simulink model "ClosedLoopPMSM"  (R2019a)
settings: Solver=FixedStepAuto  StartTime=0.0  StopTime=inf  FixedStep=Sampling_time  RelTol=1e-3
values from neighbouring files (symbols this model uses):
  DCLINK_Cap = 100e-6    (= 0.0001)    [ClosedLoopParameters.m]
  interleaving_angle_1 = 0    [ClosedLoopParameters.m]
  Rin = 1e-6    (= 1e-06)    [ClosedLoopParameters.m]
  Sampling_time = 1e-6    (= 1e-06)    [ClosedLoopParameters.m]
  Vin = Vdesired    (= 540)    [ClosedLoopParameters.m]
undefined symbols (not defined in the file or in its folder): Tload
libraries: powerlib x7, eeTransforms x4, simulink x3, powerlib_meascontrol x1
settings Model: Creator=admin  LastModifiedBy=admin

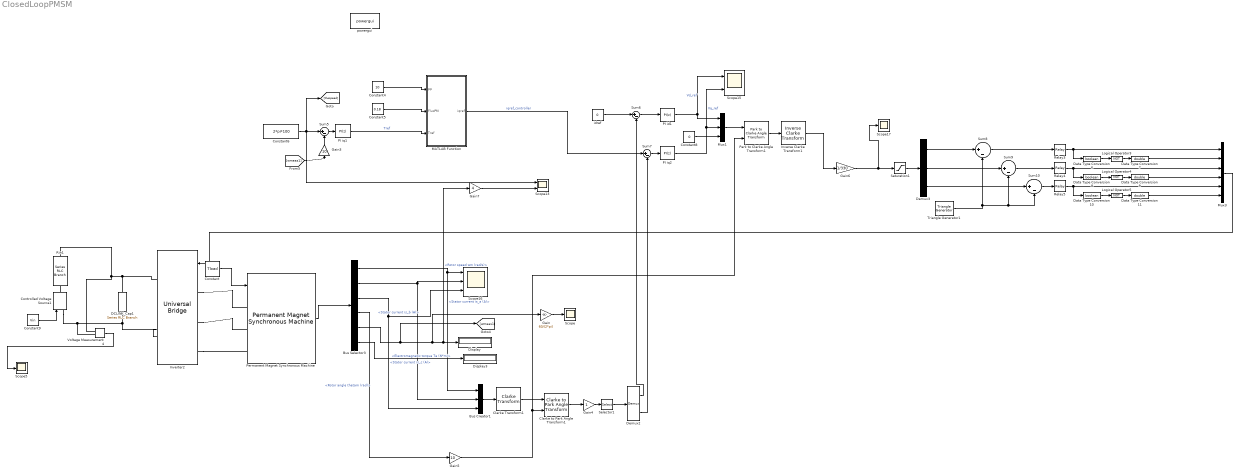
== system ClosedLoopPMSM ==
  Bus Creator1 : BusCreator  Inputs=3
  Bus Selector3 : BusSelector  OutputSignals=Stator current is_a (A),Stator current is_b (A),Stator current is_c (A),Rotor angle thetam (rad),Rotor speed wm (rad/s),Electromagnetic torque Te (N*m)
  Clarke Transform1 : eeTransforms/Clarke Transform  PowerInvariant=off
      settings: SourceProductName=Simscape Electrical  SourceProductBaseCode=PS
  Clarke to Park Angle Transform1 : eeTransforms/Clarke to Park Angle Transform  AxisAlignment=Q-axis
      settings: SourceProductName=Simscape Electrical  SourceProductBaseCode=PS
  Constant : Constant  Value=Tload
  Constant4 : Constant  Value=10
  Constant5 : Constant  Value=0.18
  Constant6 : Constant  Value=2*pi*100
  Constant8 : Constant  Value=0
  Constant9 : Constant  Value=Vin
  Controlled Voltage Source1 : powerlib/Electrical Sources/Controlled Voltage Source  Initialize=on  Source_Type=DC  Amplitude=0  Phase=0  Frequency=0  Measurements=None
      settings: SourceProductName=Simscape Electrical
  DCLINK_Cap1 : powerlib/Elements/Series RLC Branch  LConnTagsString=__new0  RConnTagsString=__new0  BranchType=C  Resistance=1  Inductance=1e-3  SetiL0=off  InitialCurrent=0  Capacitance=DCLINK_Cap  Setx0=on  InitialVoltage=540  Measurements=None
      settings: SourceProductName=Simscape Electrical
  Data Type Conversion10 : DataTypeConversion  OutDataTypeStr=boolean
  Data Type Conversion11 : DataTypeConversion  OutDataTypeStr=double
  Data Type Conversion6 : DataTypeConversion  OutDataTypeStr=boolean
  Data Type Conversion7 : DataTypeConversion  OutDataTypeStr=double
  Data Type Conversion8 : DataTypeConversion  OutDataTypeStr=boolean
  Data Type Conversion9 : DataTypeConversion  OutDataTypeStr=double
  Demux2 : Demux  Outputs=2
  Demux3 : Demux  Outputs=3
  Display : Display
  Display3 : Display
  Gain : Gain  Gain=60/(2*pi)
  Gain3 : Gain  Gain=10
  Gain4 : Gain
  Gain5 : Gain  Gain=10
  Gain6 : Gain  Gain=1/330
  Gain7 : Gain  Gain=4
  Inverse Clarke Transform1 : eeTransforms/Inverse Clarke Transform  PowerInvariant=off
      settings: SourceProductName=Simscape Electrical  SourceProductBaseCode=PS
  Inverter2 : powerlib/Power Electronics/Universal Bridge  Arms=3  SnubberResistance=1e5  SnubberCapacitance=inf  Device=IGBT / Diodes  Ron=0.65e-3  Lon=0  ForwardVoltages="[  0  0  ]"  ForwardVoltage=0  GTOparameters=[ 10e-6 , 20e-6 ]  IGBTparameters=[ 1e-6 , 2e-6 ]  Measurements=All voltages and currents  Measurements_2=None  converterType=Rectifier
      settings: SourceProductName=Simscape Electrical
  Logical Operator3 : Logic  Operator=NOT  AllPortsSameDT=off  OutDataTypeStr=boolean
  Logical Operator4 : Logic  Operator=NOT  AllPortsSameDT=off  OutDataTypeStr=boolean
  Logical Operator5 : Logic  Operator=NOT  AllPortsSameDT=off  OutDataTypeStr=boolean
  MATLAB Function : MATLAB Function  TreatAsAtomicUnit=on
  Mux1 : Mux  Inputs=3
  Mux3 : Mux  Inputs=6
  PI id1 : simulink/Continuous/PID Controller  Controller=PI  Form=Parallel  TimeDomain=Discrete-time  SampleTime=-1  IntegratorMethod=Forward Euler  FilterMethod=Forward Euler  ControllerParametersSource=internal  P=0.5  I=5  D=0  UseFilter=on  N=100  TunerSelectOption=Transfer Function Based (PID Tuner App)  InitialConditionSource=internal  InitialConditionForIntegrator=0  InitialConditionForFilter=0  DifferentiatorICPrevScaledInput=0  ExternalReset=none  TrackingMode=off  Kt=1  LimitOutput=off  UpperSaturationLimit=inf  LowerSaturationLimit=-inf  LinearizeAsGain=on  AntiWindupMode=none  Kb=1  POutMin=[]  POutMax=[]  IOutMin=[]  IOutMax=[]  DOutMin=[]  DOutMax=[]  NOutMin=[]  NOutMax=[]  SumOutMin=[]  SumOutMax=[]  SaturationOutMin=[]  SaturationOutMax=[]  PParamMin=[]  PParamMax=[]  IParamMin=[]  IParamMax=[]  DParamMin=[]  DParamMax=[]  NParamMin=[]  NParamMax=[]  KbParamMin=[]  KbParamMax=[]  KtParamMin=[]  KtParamMax=[]  KbOutMin=[]  KbOutMax=[]  KtOutMin=[]  KtOutMax=[]  IntegratorOutMin=[]  IntegratorOutMax=[]  FilterOutMin=[]  FilterOutMax=[]  SumI1OutMin=[]  SumI1OutMax=[]  SumI2OutMin=[]  SumI2OutMax=[]  SumI3OutMin=[]  SumI3OutMax=[]  SumI4OutMin=[]  SumI4OutMax=[]  SumDOutMin=[]  SumDOutMax=[]  DifferentiatorOutMin=[]  DifferentiatorOutMax=[]  FilterDiffOutCoefMin=[]  FilterDiffOutCoefMax=[]  ReciprocalOutMin=[]  ReciprocalOutMax=[]  SumDenOutMin=[]  SumDenOutMax=[]  SumNumOutMin=[]  SumNumOutMax=[]  DivideOutMin=[]  DivideOutMax=[]  IntegratorContinuousStateAttributes=''  IntegratorStateMustResolveToSignalObject=off  IntegratorRTWStateStorageClass=Auto  FilterContinuousStateAttributes=''  FilterStateMustResolveToSignalObject=off  FilterRTWStateStorageClass=Auto  ParallelPVariant=InternalParameters  IdealPVariant=Disabled  IVariant=InternalParameters  DVariant=Disabled  IntegratorVariant=Discrete  SatVariant=Disabled  AWVariant=Passthrough  PCopyVariant=Disabled  TRVariant=Disabled  FdbkBlocksVariant=Forward  IdealPFdbkVariant=Disabled  SatFdbkVariant=Disabled  DerivativeFilterVariant=Disabled  NVariant=Disabled  NCopyVariant=Disabled_SignalSpec  FilterICVariant=Disabled  IntegratorICVariant=InternalICs  ExternalResetVariant=Disabled  TRSumVariant=Passthrough  SumFdbkVariant=Disabled  SumVariant=Sum_PI
  PI iq1 : simulink/Continuous/PID Controller  Controller=PI  Form=Parallel  TimeDomain=Discrete-time  SampleTime=-1  IntegratorMethod=Forward Euler  FilterMethod=Forward Euler  ControllerParametersSource=internal  P=100  I=10  D=0  UseFilter=on  N=100  TunerSelectOption=Transfer Function Based (PID Tuner App)  InitialConditionSource=internal  InitialConditionForIntegrator=0  InitialConditionForFilter=0  DifferentiatorICPrevScaledInput=0  ExternalReset=none  TrackingMode=off  Kt=1  LimitOutput=off  UpperSaturationLimit=inf  LowerSaturationLimit=-inf  LinearizeAsGain=on  AntiWindupMode=none  Kb=1  POutMin=[]  POutMax=[]  IOutMin=[]  IOutMax=[]  DOutMin=[]  DOutMax=[]  NOutMin=[]  NOutMax=[]  SumOutMin=[]  SumOutMax=[]  SaturationOutMin=[]  SaturationOutMax=[]  PParamMin=[]  PParamMax=[]  IParamMin=[]  IParamMax=[]  DParamMin=[]  DParamMax=[]  NParamMin=[]  NParamMax=[]  KbParamMin=[]  KbParamMax=[]  KtParamMin=[]  KtParamMax=[]  KbOutMin=[]  KbOutMax=[]  KtOutMin=[]  KtOutMax=[]  IntegratorOutMin=[]  IntegratorOutMax=[]  FilterOutMin=[]  FilterOutMax=[]  SumI1OutMin=[]  SumI1OutMax=[]  SumI2OutMin=[]  SumI2OutMax=[]  SumI3OutMin=[]  SumI3OutMax=[]  SumI4OutMin=[]  SumI4OutMax=[]  SumDOutMin=[]  SumDOutMax=[]  DifferentiatorOutMin=[]  DifferentiatorOutMax=[]  FilterDiffOutCoefMin=[]  FilterDiffOutCoefMax=[]  ReciprocalOutMin=[]  ReciprocalOutMax=[]  SumDenOutMin=[]  SumDenOutMax=[]  SumNumOutMin=[]  SumNumOutMax=[]  DivideOutMin=[]  DivideOutMax=[]  IntegratorContinuousStateAttributes=''  IntegratorStateMustResolveToSignalObject=off  IntegratorRTWStateStorageClass=Auto  FilterContinuousStateAttributes=''  FilterStateMustResolveToSignalObject=off  FilterRTWStateStorageClass=Auto  ParallelPVariant=InternalParameters  IdealPVariant=Disabled  IVariant=InternalParameters  DVariant=Disabled  IntegratorVariant=Discrete  SatVariant=Disabled  AWVariant=Passthrough  PCopyVariant=Disabled  TRVariant=Disabled  FdbkBlocksVariant=Forward  IdealPFdbkVariant=Disabled  SatFdbkVariant=Disabled  DerivativeFilterVariant=Disabled  NVariant=Disabled  NCopyVariant=Disabled_SignalSpec  FilterICVariant=Disabled  IntegratorICVariant=InternalICs  ExternalResetVariant=Disabled  TRSumVariant=Passthrough  SumFdbkVariant=Disabled  SumVariant=Sum_PI
  PI iq2 : simulink/Continuous/PID Controller  Controller=PI  Form=Parallel  TimeDomain=Discrete-time  SampleTime=-1  IntegratorMethod=Forward Euler  FilterMethod=Forward Euler  ControllerParametersSource=internal  P=0.5  I=5  D=0  UseFilter=on  N=100  TunerSelectOption=Transfer Function Based (PID Tuner App)  InitialConditionSource=internal  InitialConditionForIntegrator=0  InitialConditionForFilter=0  DifferentiatorICPrevScaledInput=0  ExternalReset=none  TrackingMode=off  Kt=1  LimitOutput=off  UpperSaturationLimit=inf  LowerSaturationLimit=-inf  LinearizeAsGain=on  AntiWindupMode=none  Kb=1  POutMin=[]  POutMax=[]  IOutMin=[]  IOutMax=[]  DOutMin=[]  DOutMax=[]  NOutMin=[]  NOutMax=[]  SumOutMin=[]  SumOutMax=[]  SaturationOutMin=[]  SaturationOutMax=[]  PParamMin=[]  PParamMax=[]  IParamMin=[]  IParamMax=[]  DParamMin=[]  DParamMax=[]  NParamMin=[]  NParamMax=[]  KbParamMin=[]  KbParamMax=[]  KtParamMin=[]  KtParamMax=[]  KbOutMin=[]  KbOutMax=[]  KtOutMin=[]  KtOutMax=[]  IntegratorOutMin=[]  IntegratorOutMax=[]  FilterOutMin=[]  FilterOutMax=[]  SumI1OutMin=[]  SumI1OutMax=[]  SumI2OutMin=[]  SumI2OutMax=[]  SumI3OutMin=[]  SumI3OutMax=[]  SumI4OutMin=[]  SumI4OutMax=[]  SumDOutMin=[]  SumDOutMax=[]  DifferentiatorOutMin=[]  DifferentiatorOutMax=[]  FilterDiffOutCoefMin=[]  FilterDiffOutCoefMax=[]  ReciprocalOutMin=[]  ReciprocalOutMax=[]  SumDenOutMin=[]  SumDenOutMax=[]  SumNumOutMin=[]  SumNumOutMax=[]  DivideOutMin=[]  DivideOutMax=[]  IntegratorContinuousStateAttributes=''  IntegratorStateMustResolveToSignalObject=off  IntegratorRTWStateStorageClass=Auto  FilterContinuousStateAttributes=''  FilterStateMustResolveToSignalObject=off  FilterRTWStateStorageClass=Auto  ParallelPVariant=InternalParameters  IdealPVariant=Disabled  IVariant=InternalParameters  DVariant=Disabled  IntegratorVariant=Discrete  SatVariant=Disabled  AWVariant=Passthrough  PCopyVariant=Disabled  TRVariant=Disabled  FdbkBlocksVariant=Forward  IdealPFdbkVariant=Disabled  SatFdbkVariant=Disabled  DerivativeFilterVariant=Disabled  NVariant=Disabled  NCopyVariant=Disabled_SignalSpec  FilterICVariant=Disabled  IntegratorICVariant=InternalICs  ExternalResetVariant=Disabled  TRSumVariant=Passthrough  SumFdbkVariant=Disabled  SumVariant=Sum_PI
  Park to Clarke Angle Transform1 : eeTransforms/Park to Clarke Angle Transform  AxisAlignment=Q-axis
      settings: SourceProductName=Simscape Electrical  SourceProductBaseCode=PS
  Permanent Magnet Synchronous Machine : powerlib/Machines/Permanent Magnet Synchronous Machine  NbPhases=3  FluxDistribution=Sinusoidal  RotorType=Salient-pole  MechanicalLoad=Torque Tm  PresetModel=No  ShowDetailedParameters=on  MeasurementBus=off  Resistance=0.320  Inductance=8.5e-3  dqInductances=[3.1e-3,3.6e-3]  La=0.000395  MachineConstant=Flux linkage established by magnets (V.s)  Flux=0.18  VoltageCst=326.4839  TorqueCst=2.7  Flat=120  Mechanical=[0.0027 0.0004924 10 0]  PolePairs=4  InitialConditions=[0,0, 0,0]  InitialConditions5ph=[0 0 0 0 0 0]  TsPowergui=0  TsBlock=-1  RefAngle=90 degrees behind phase A axis (modified Park)
  Relay3 : Relay
  Relay4 : Relay
  Relay5 : Relay
  Rin1 : powerlib/Elements/Series RLC Branch  LConnTagsString=__new0  RConnTagsString=__new0  BranchType=R  Resistance=Rin  Inductance=1e-3  SetiL0=off  InitialCurrent=0  Capacitance=1000e-6  Setx0=off  InitialVoltage=0  Measurements=None
      settings: SourceProductName=Simscape Electrical
  Saturation1 : Saturate  UpperLimit=1  LowerLimit=-1
  Scope : Scope
  Scope13 : Scope  NumInputPorts=2
  Scope15 : Scope  NumInputPorts=2
  Scope16 : Scope  NumInputPorts=3
  Scope17 : Scope
  Scope5 : Scope
  Selector1 : Selector  InputPortWidth=3  IndexOptions=Index vector (dialog)  Indices=[1 2]  OutputSizes=1
  Sum{5..10} (6 alike) : Sum  Inputs=|+-
  Triangle Generator1 : powerlib_meascontrol/Pulse & Signal Generators/Triangle Generator  Freq=sw_frequency  Phase=interleaving_angle_1  Ts=Sampling_time
      settings: SourceProductName=Simscape Electrical
  Voltage Measurement4 : powerlib/Measurements/Voltage Measurement  PhasorSimulation=off  OutputType=Complex  PSBequivalent=0
      settings: SourceProductName=Simscape Electrical
  idref : Constant  Value=0
  powergui : powerlib/powergui  Priority=1  SimulationMode=Discrete  SampleTime=Sampling_time  frequency=60  Iterations=50  frequencyindice=0  Pbase=100e6  ErrMax=1e-4  UnitsV=kV  UnitsW=MW  buscounter=0  FunctionMessages=off  echomessages=off  EnableUseOfTLC=off  CurrentSourceSwitches=off  DisableSnubberDevices=off  DisableRonSwitches=off  DisableVfSwitches=off  DisplayEquations=off  AutomaticDiscreteSolvers=off  SolverType=Tustin/Backward Euler (TBE)  Interpol=off  ExternalGateDelay=off  methode=off  Ts=100  x0status=blocks  SPID=on  SwTol=0  HookPort=off  NonlinearTolerance=0  nMaxIteration=15  ContinueOnMaxIteration=off  RestoreLinks=warning  ResistiveCurrentMeasurement=off  Frange=[0:2:500]  Ylog=off  Xlog=on  ShowGrid=off  save=off  variable=ZData  structure=0  ZoomFFT=off  StartTime=0.0  cycles=1  DisplayStyle=1  fundamental=60  FreqAxis=off  MaxFrequency=1000  frequencyindicesteady=1  RmsSteady=1  display=off
      settings: SourceProductName=Simscape Electrical
  wires:
  Logical Operator5/1 -> Data Type Conversion11/1
  Bus Selector3/2 -> Bus Creator1/2, Scope16/2  "<Stator current is_b (A)>"
  Bus Creator1/1 -> Clarke Transform1/1
  Constant9/1 -> Controlled Voltage Source1/1
  Clarke to Park Angle Transform1/1 -> Gain4/1
  Selector1/1 -> Demux2/1
  Inverse Clarke Transform1/1 -> Gain6/1
  [wmeas1] -> Gain3/1
  PI iq2/1 -> Scope15/2, Mux1/2  "Vq_ref"
  PI iq1/1 -> MATLAB Function/3(Tref)  "Tref"
  PI id1/1 -> Scope15/1, Mux1/1  "Vd_ref"
  Sum6/1 -> PI id1/1
  Constant8/1 -> Mux1/3
  Mux1/1 -> Park to Clarke Angle Transform1/1
  Gain5/1 -> Park to Clarke Angle Transform1/2, Clarke to Park Angle Transform1/2
  Gain3/1 -> Sum5/2
  Constant5/1 -> MATLAB Function/2(FluxPM)
  Constant4/1 -> MATLAB Function/1(pp)
  Clarke Transform1/1 -> Clarke to Park Angle Transform1/1
  Saturation1/1 -> Demux3/1
  Gain7/1 -> Scope13/2
  Constant6/1 -> [thespeed], Scope13/1, Sum5/1
  Relay5/1 -> Mux3/5, Data Type Conversion10/1
  Bus Selector3/5 -> [wmeas1], Gain/1, Gain7/1, Display/1  "<Rotor speed wm (rad/s)>"
  Demux2/1 -> Sum6/2
  Sum10/1 -> Relay5/1
  Data Type Conversion7/1 -> Mux3/2
  Mux3/1 -> Inverter2/1
  Triangle Generator1/1 -> Sum8/2, Sum10/2, Sum9/2
  Gain4/1 -> Selector1/1
  Bus Selector3/4 -> Gain5/1  "<Rotor angle thetam (rad)>"
  Demux3/2 -> Sum9/1
  Logical Operator4/1 -> Data Type Conversion9/1
  idref/1 -> Sum6/1
  Sum8/1 -> Relay3/1
  Gain6/1 -> Scope17/1, Saturation1/1
  Bus Selector3/1 -> Scope16/1, Bus Creator1/1  "<Stator current is_a (A)>"
  Logical Operator3/1 -> Data Type Conversion7/1
  Data Type Conversion8/1 -> Logical Operator4/1
  Data Type Conversion11/1 -> Mux3/6
  Permanent Magnet Synchronous Machine/1 -> Bus Selector3/1
  Relay3/1 -> Mux3/1, Data Type Conversion6/1
  Data Type Conversion9/1 -> Mux3/4
  MATLAB Function/1(iqref) -> Sum7/1  "iqref_controller"
  Park to Clarke Angle Transform1/1 -> Inverse Clarke Transform1/1
  Sum5/1 -> PI iq1/1
  Demux3/1 -> Sum8/1
  Data Type Conversion10/1 -> Logical Operator5/1
  Demux3/3 -> Sum10/1
  Sum7/1 -> PI iq2/1
  Sum9/1 -> Relay4/1
  Demux2/2 -> Sum7/2
  Data Type Conversion6/1 -> Logical Operator3/1
  Bus Selector3/3 -> Bus Creator1/3, Scope16/3  "<Stator current is_c (A)>"
  Voltage Measurement4/1 -> Scope5/1
  Relay4/1 -> Mux3/3, Data Type Conversion8/1
  Bus Selector3/6 -> Display3/1  "<Electromagnetic torque Te (N*m)>"
  Constant/1 -> Permanent Magnet Synchronous Machine/1
  Gain/1 -> Scope/1
  connections:
  Controlled Voltage Source1/LConn1 -- Voltage Measurement4/LConn2 -- Inverter2/RConn2 -- DCLINK_Cap1/RConn1
  Voltage Measurement4/LConn1 -- DCLINK_Cap1/LConn1 -- Inverter2/RConn1 -- Rin1/LConn1
  Inverter2/LConn3 -- Permanent Magnet Synchronous Machine/LConn3
  Inverter2/LConn2 -- Permanent Magnet Synchronous Machine/LConn2
  Controlled Voltage Source1/RConn1 -- Rin1/RConn1
  Inverter2/LConn1 -- Permanent Magnet Synchronous Machine/LConn1

== matlab function ClosedLoopPMSM/MATLAB Function ==
  data: pp input; iqref output; FluxPM input; Tref input
function iqref = fcn(pp,FluxPM,Tref)

iqref = Tref/((3/2)*FluxPM*pp);
